simulink model "Flyback_snubber"  (R2016a)
settings: Solver=VariableStepAuto  StartTime=0.0  StopTime=0.1  RelTol=1e-3
libraries: powerlib x18
settings Model: Creator=Mac  LastModifiedBy=Hp

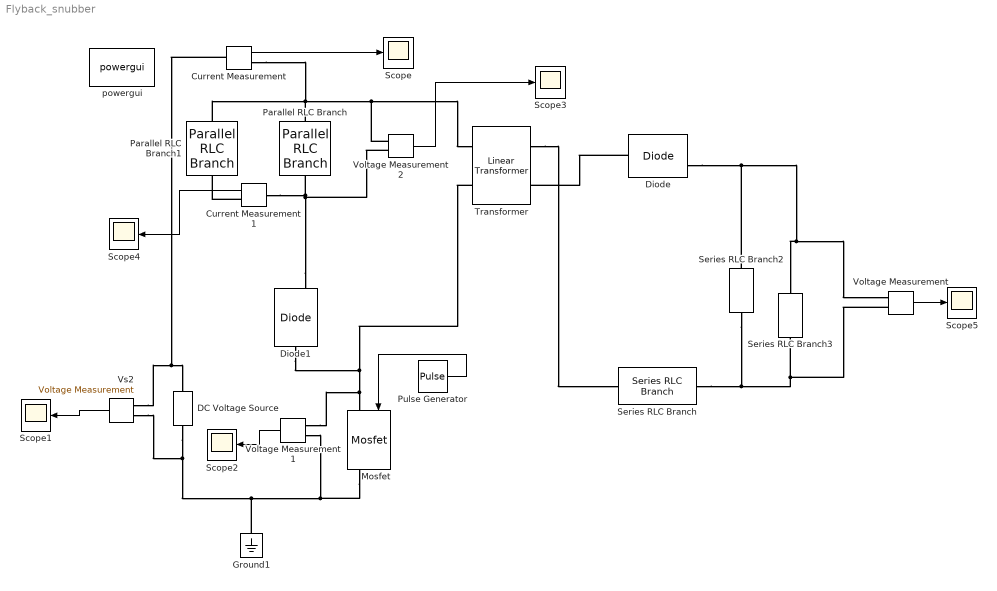
== system Flyback_snubber ==
  Current Measurement : powerlib/Measurements/Current Measurement  PhasorSimulation=off  OutputType=Complex  PSBequivalent=0
  Current Measurement1 : powerlib/Measurements/Current Measurement  PhasorSimulation=off  OutputType=Complex  PSBequivalent=0
  DC Voltage Source : powerlib/Electrical Sources/DC Voltage Source  Amplitude=12  Measurements=None
  Diode : powerlib/Power Electronics/Diode  Ron=0.001  Lon=0  Vf=0.8  IC=0  UseSnubber=off  Rs=500  Cs=250e-9  Measurements=on
  Diode1 : powerlib/Power Electronics/Diode  Ron=0.001  Lon=0  Vf=0.8  IC=0  UseSnubber=off  Rs=500  Cs=250e-9  Measurements=on
  Ground1 : powerlib/Elements/Ground  LConnTagsString=a
  Mosfet : powerlib/Power Electronics/Mosfet  Ron=0.00001  Lon=0  Rd=0.01  Vfd=0  IC=0  Rs=0  Cs=0  Measurements=on
  Parallel RLC Branch : powerlib/Elements/Parallel RLC Branch  LConnTagsString=a  RConnTagsString=__new0  BranchType=C  Resistance=50  Inductance=1e-3  SetiL0=off  InitialCurrent=0  Capacitance=10e-6  Setx0=off  InitialVoltage=0  Measurements=None
  Parallel RLC Branch1 : powerlib/Elements/Parallel RLC Branch  LConnTagsString=a  RConnTagsString=__new0  BranchType=R  Resistance=1000  Inductance=1e-3  SetiL0=off  InitialCurrent=0  Capacitance=1e-6  Setx0=off  InitialVoltage=0  Measurements=None
  Pulse Generator : DiscretePulseGenerator  PulseType=Time based  Period=2e-5  PulseWidth=60
  Scope{,1..5} (6 alike) : Scope
  Series RLC Branch : powerlib/Elements/Series RLC Branch  LConnTagsString=__new0  RConnTagsString=__new0  BranchType=R  Resistance=0.000001  Inductance=1e-3  SetiL0=off  InitialCurrent=0  Capacitance=1e-6  Setx0=off  InitialVoltage=0  Measurements=None
  Series RLC Branch2 : powerlib/Elements/Series RLC Branch  LConnTagsString=__new0  RConnTagsString=__new0  BranchType=C  Resistance=25.6  Inductance=200e-3  SetiL0=off  InitialCurrent=0  Capacitance=100e-6  Setx0=off  InitialVoltage=0  Measurements=Branch voltage
  Series RLC Branch3 : powerlib/Elements/Series RLC Branch  LConnTagsString=__new0  RConnTagsString=__new0  BranchType=R  Resistance=25.6  Inductance=200e-3  SetiL0=off  InitialCurrent=0  Capacitance=1e-6  Setx0=off  InitialVoltage=0  Measurements=Branch voltage
  Transformer : powerlib/Elements/Linear Transformer  UNITS=SI  NominalPower=[ 1000 50e3 ]  winding1=[500 0.147 600e-9]  winding2=[900 0 0]  ThreeWindings=off  winding3=[3.15e+05 315.06 8.8673e-08]  RmLm=[100000 6.27e-6]  Measurements=All voltages and currents  DataType=on
  Voltage Measurement : powerlib/Measurements/Voltage Measurement  PhasorSimulation=off  OutputType=Complex  PSBequivalent=0
  Voltage Measurement1 : powerlib/Measurements/Voltage Measurement  PhasorSimulation=off  OutputType=Complex  PSBequivalent=0
  Voltage Measurement2 : powerlib/Measurements/Voltage Measurement  PhasorSimulation=off  OutputType=Complex  PSBequivalent=0
  Vs2 : powerlib/Measurements/Voltage Measurement  PhasorSimulation=off  OutputType=Complex  PSBequivalent=0
  "powergui " : powerlib/powergui  Priority=1  SimulationMode=Discrete  SolverType=Tustin/Backward Euler (TBE)  SampleTime=1e-7  frequency=60  SPID=on  DisableSnubberDevices=off  DisableRonSwitches=on  DisableVfSwitches=on  SwTol=0  DisplayEquations=off  Interpol=off  ExternalGateDelay=off  methode=off  Ts=10  FunctionMessages=off  echomessages=off  HookPort=off  EnableUseOfTLC=off  x0status=blocks  frequencyindice=0  Pbase=100e6  ErrMax=1e-4  Iterations=50  UnitsV=kV  UnitsW=MW  buscounter=0  RestoreLinks=warning  ResistiveCurrentMeasurement=off  Frange=[0:2:500]  Ylog=off  Xlog=on  ShowGrid=off  save=off  variable=ZData  structure=0  ZoomFFT=off  StartTime=0.0  cycles=1  DisplayStyle=1  fundamental=60  FreqAxis=off  MaxFrequency=1000  frequencyindicesteady=1  RmsSteady=1  display=off
  wires:
  Voltage Measurement/1 -> Scope5/1
  Vs2/1 -> Scope1/1
  Pulse Generator/1 -> Mosfet/1
  Current Measurement/1 -> Scope/1
  Voltage Measurement1/1 -> Scope2/1
  Voltage Measurement2/1 -> Scope3/1
  Current Measurement1/1 -> Scope4/1
  connections:
  Vs2/LConn2 -- DC Voltage Source/LConn1 -- Ground1/LConn1 -- Mosfet/RConn1 -- Voltage Measurement1/LConn2
  Series RLC Branch2/LConn1 -- Diode/RConn1 -- Voltage Measurement/LConn1 -- Series RLC Branch3/LConn1
  Transformer/LConn2 -- Diode1/LConn1 -- Voltage Measurement1/LConn1 -- Mosfet/LConn1
  Vs2/LConn1 -- Current Measurement/LConn1 -- DC Voltage Source/RConn1
  Diode/LConn1 -- Transformer/RConn2
  Voltage Measurement/LConn2 -- Series RLC Branch/RConn1 -- Series RLC Branch2/RConn1 -- Series RLC Branch3/RConn1
  Current Measurement/RConn1 -- Parallel RLC Branch1/LConn1 -- Parallel RLC Branch/LConn1 -- Voltage Measurement2/LConn1 -- Transformer/LConn1
  Transformer/RConn1 -- Series RLC Branch/LConn1
  Diode1/RConn1 -- Current Measurement1/LConn1 -- Parallel RLC Branch/RConn1 -- Voltage Measurement2/LConn2
  Current Measurement1/RConn1 -- Parallel RLC Branch1/RConn1
